simulink model "bai28"  (R2016a)
settings: Solver=VariableStepAuto  StartTime=0.0  StopTime=10.0  RelTol=1e-3
settings Model: Creator=HP  LastModifiedBy=HP

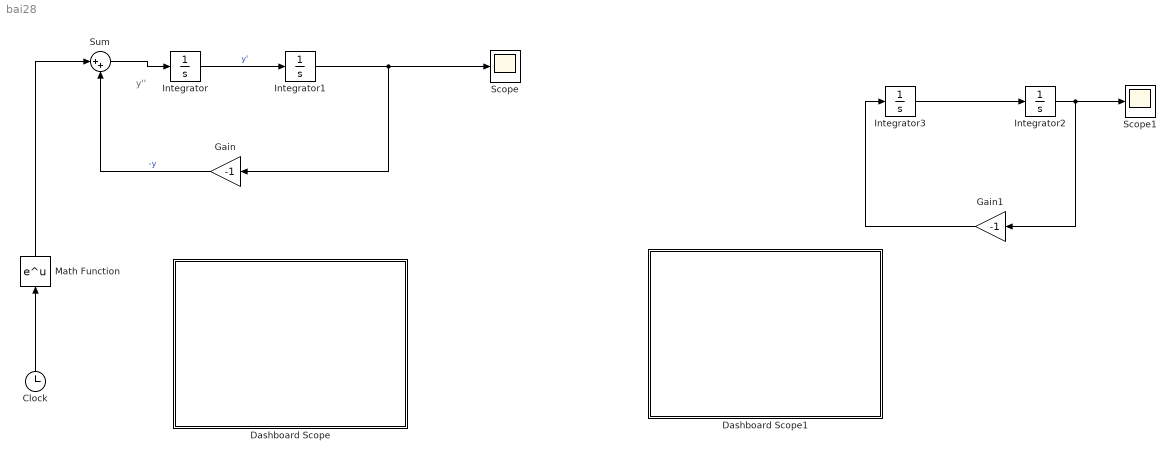
== system bai28 ==
  note: y''
  Clock : Clock
  Dashboard Scope : Subsystem  DialogController=hmiCreateDDGDialog  IsWebBlock=on  mask(MWDashboardBlock){webBlockId=9a679459-dfb4-481c-91f3-1b0390eefb46, webBlockType=sdiscope, ShowInitialText=on, HMISrcModelName=bai28}
      mask prompts: webBlockId "WebBlock Id"; webBlockType "WebBlock Type"; HMISrcModelName "Source Model"
      mask Help: helpview([docroot '/mapfiles/simulink.map'], 'hmi_scope')
      mask Display:
      | if strcmp(get_param(bdroot(gcb),'BlockDiagramType'), 'library')
      |     image([(matlabroot) '/toolbox/simulink/hmi/icons/DashboardScope.png']);
      | end
  Dashboard Scope1 : Subsystem  DialogController=hmiCreateDDGDialog  IsWebBlock=on  mask(MWDashboardBlock){webBlockId=2cef69d5-53f7-4686-91e6-5204d8786a04, webBlockType=sdiscope, ShowInitialText=on, HMISrcModelName=bai28}
      mask prompts: webBlockId "WebBlock Id"; webBlockType "WebBlock Type"; HMISrcModelName "Source Model"
      mask Help: helpview([docroot '/mapfiles/simulink.map'], 'hmi_scope')
      mask Display:
      | if strcmp(get_param(bdroot(gcb),'BlockDiagramType'), 'library')
      |     image([(matlabroot) '/toolbox/simulink/hmi/icons/DashboardScope.png']);
      | end
  Gain : Gain  Gain=-1
  Gain1 : Gain  Gain=-1
  Integrator : Integrator
  Integrator1 : Integrator  InitialCondition=1
  Integrator2 : Integrator  InitialCondition=1
  Integrator3 : Integrator
  Math Function : Math  SaturateOnIntegerOverflow=on
  Scope : Scope
  Scope1 : Scope
  Sum : Sum  Inputs=|++
  wires:
  Integrator/1 -> Integrator1/1  "y'"
  Integrator1/1 -> Scope/1, Gain/1
  Gain/1 -> Sum/2  "-y"
  Clock/1 -> Math Function/1
  Math Function/1 -> Sum/1
  Sum/1 -> Integrator/1
  Integrator3/1 -> Integrator2/1
  Gain1/1 -> Integrator3/1
  Integrator2/1 -> Scope1/1, Gain1/1

== system bai28/Dashboard Scope ==

== system bai28/Dashboard Scope1 ==
